simulink model "LLM_Testing"  (R2025b)
settings: Solver=ode8  StartTime=0.0  StopTime=1000  FixedStep=0.0001  RelTol=1e-3
libraries: simulink_extras x2, aerolibactuator x1
settings Model: Creator=jonno  LastModifiedBy=jonno

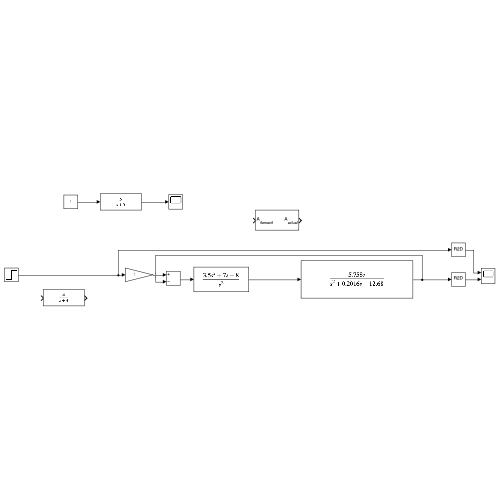
[thumbnail: Simulink's stored preview of the top-level diagram]
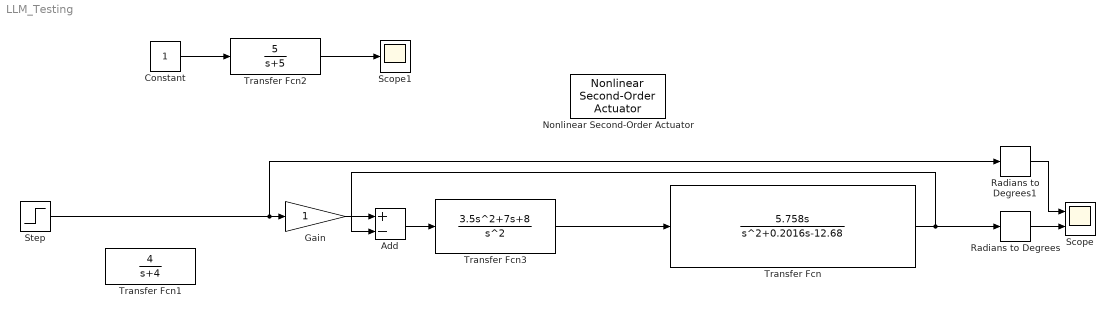
== system LLM_Testing ==
  Add : Sum  Inputs=+-
  Constant : Constant
  Gain : Gain
  Nonlinear Second-Order Actuator : aerolibactuator/Nonlinear Second-Order Actuator  wn_fin=62  z_fin=0.707  fin_max=100000  fin_min=-100000  fin_maxrate=100000  fin_act_0=0  fin_act_vel=0
  Radians to Degrees : simulink_extras/Transformations/Radians to Degrees
  Radians to Degrees1 : simulink_extras/Transformations/Radians to Degrees
  Scope : Scope  NumInputPorts=2
      settings: ActiveDisplayYMinimum=-0.16258352467725984  ActiveDisplayYMaximum=1.4632517220953387
  Scope1 : Scope
      settings: ActiveDisplayYMinimum=-1  ActiveDisplayYMaximum=1
  Step : Step  Time=0  After=deg2rad(1)  SampleTime=0
  Transfer Fcn : TransferFcn  Numerator=[5.758 0]  Denominator=[1 0.2016 -12.68]
  Transfer Fcn1 : TransferFcn  Numerator=[4]  Denominator=[1 4]
  Transfer Fcn2 : TransferFcn  Numerator=[5]  Denominator=[1 5]
  Transfer Fcn3 : TransferFcn  Numerator=[3.5 7 8]  Denominator=[1 0 0]
  wires:
  Transfer Fcn/1 -> Add/2, Radians to Degrees/1
  Radians to Degrees/1 -> Scope/2
  Add/1 -> Transfer Fcn3/1
  Step/1 -> Radians to Degrees1/1, Gain/1
  Radians to Degrees1/1 -> Scope/1
  Gain/1 -> Add/1
  Constant/1 -> Transfer Fcn2/1
  Transfer Fcn2/1 -> Scope1/1
  Transfer Fcn3/1 -> Transfer Fcn/1
